simulink model "Sim_normboundsystem_simtest"  (Simulink 7.3)
settings: Solver=ode45  StartTime=0.0  StopTime=10  RelTol=1e-3
settings Model: Creator=MD710  LastModifiedBy=MD710
settings DebuggingCC: SaveWithParameterizedLinksMsg=none  MultiTaskDSMMsg=warning  MultiTaskCondExecSysMsg=none  FcnCallInpInsideContextMsg=Enable All  StrictBusMsg=None
settings HardwareCC: TargetHWDeviceType=32-bit Generic
settings RTWCC: IncludeERTFirstTime=on
settings GRTTargetCC: TargetFcnLib=ansi_tfl_tmw.mat

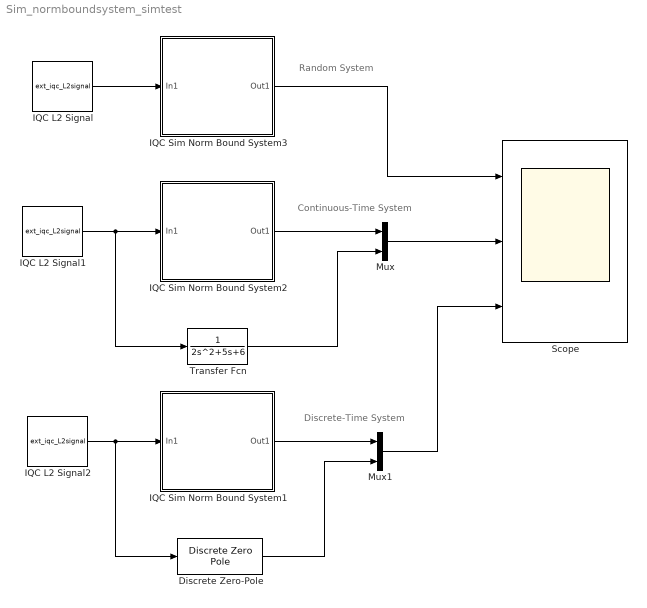
== system Sim_normboundsystem_simtest ==
  note: Random System
  note: Continuous-Time System
  note: Discrete-Time System
  Discrete Zero-Pole : DiscreteZeroPole  Zeros=[]  Poles=[0.3 -0.5]  Gain=1
  IQC L2 Signal : M-S-Function  FunctionName=ext_iqc_L2signal  Parameters=sig_size,sam_time,sig_type,tru_time,sig_amp,sig_fre,user_cus  mask(IQC L2 signal(ver:0.1)){sig_size=1, sam_time=0, sig_type=Sine wave, tru_time=10, sig_amp=1, sig_fre=1, user_cus='2*exp(3*t)'}
      mask prompts: sig_size "Signal Dimension:(Default: 1)"; sam_time "Sample Time:(Default: 0)"; sig_type "Signal Type:"; tru_time "Truncation Time:"; sig_amp "Maximum Amplitude:"; sig_fre "Frequency:"; user_cus "Custom:"
      mask help:
      | Important:
      | In IQC procedure step (as commond iqc_gain_tbx, the task is get
      | L2 gain value), regardless of the user to choose which option (ex sine...),
      | here regarded as generalized L2 signal.
      mask StyleString: edit,edit,popup(Step|Square wave|Sine wave|Custom|Random|External),edit,edit,edit,edit
      mask CallbackString: ||iqc_block_cho(gcb,'L2signal_type')||||
      mask TabNameString: Main,Main,Simulation,Simulation,Simulation,Simulation,Simulation
      mask Display: plot(0:0.1:10,[sin(0:0.1:6.2) zeros(1,38)])
  IQC L2 Signal1 : M-S-Function  FunctionName=ext_iqc_L2signal  Parameters=sig_size,sam_time,sig_type,tru_time,sig_amp,sig_fre,user_cus  mask(IQC L2 signal(ver:0.1)){sig_size=1, sam_time=0, sig_type=Sine wave, tru_time=10, sig_amp=1, sig_fre=1, user_cus='2*exp(3*t)'}
      mask prompts: sig_size "Signal Dimension:(Default: 1)"; sam_time "Sample Time:(Default: 0)"; sig_type "Signal Type:"; tru_time "Truncation Time:"; sig_amp "Maximum Amplitude:"; sig_fre "Frequency:"; user_cus "Custom:"
      mask help:
      | Important:
      | In IQC procedure step (as commond iqc_gain_tbx, the task is get
      | L2 gain value), regardless of the user to choose which option (ex sine...),
      | here regarded as generalized L2 signal.
      mask StyleString: edit,edit,popup(Step|Square wave|Sine wave|Custom|Random|External),edit,edit,edit,edit
      mask CallbackString: ||iqc_block_cho(gcb,'L2signal_type')||||
      mask TabNameString: Main,Main,Simulation,Simulation,Simulation,Simulation,Simulation
      mask Display: plot(0:0.1:10,[sin(0:0.1:6.2) zeros(1,38)])
  IQC L2 Signal2 : M-S-Function  FunctionName=ext_iqc_L2signal  Parameters=sig_size,sam_time,sig_type,tru_time,sig_amp,sig_fre,user_cus  mask(IQC L2 signal(ver:0.1)){sig_size=1, sam_time=1, sig_type=Sine wave, tru_time=10, sig_amp=1, sig_fre=1, user_cus='2*exp(3*t)'}
      mask prompts: sig_size "Signal Dimension:(Default: 1)"; sam_time "Sample Time:(Default: 0)"; sig_type "Signal Type:"; tru_time "Truncation Time:"; sig_amp "Maximum Amplitude:"; sig_fre "Frequency:"; user_cus "Custom:"
      mask help:
      | Important:
      | In IQC procedure step (as commond iqc_gain_tbx, the task is get
      | L2 gain value), regardless of the user to choose which option (ex sine...),
      | here regarded as generalized L2 signal.
      mask StyleString: edit,edit,popup(Step|Square wave|Sine wave|Custom|Random|External),edit,edit,edit,edit
      mask CallbackString: ||iqc_block_cho(gcb,'L2signal_type')||||
      mask TabNameString: Main,Main,Simulation,Simulation,Simulation,Simulation,Simulation
      mask Display: plot(0:0.1:10,[sin(0:0.1:6.2) zeros(1,38)])
  IQC Sim Norm Bound System1 : Subsystem  mask(IQC Sim Norm Bound System(ver:0.1)){sou_sys=Custom, num_inp=1, num_out=1, num_sta=3, upp_bou=1, sam_tim=1, cus='1/((z-0.3)*(z+0.5))', var_nam='', iqc1=on, iqc1_pole=[4], iqc1_out='', iqc2=on, lis_rel='out==iqc_ltigain(in)', swsystemtype=0, A=0, B=0, C=0, D=0, newsam_tim=0}
      mask prompts: sou_sys "Source of the system:(Default: Random)"; num_inp "The Number of Input:(Default: 1)"; num_out "The Number of Output:(Default: 1)"; num_sta "The Number of States:(Default: 1)"; upp_bou "Upper Bound of the Hinf-Norm:(default: 1)"; sam_tim "Sample Time:(Default: 0)"; cus "Custom: (Default: '1/(s+1)' or '1/(z+0.5)')"; var_nam "Variable Name:(Default: empty)"; iqc1 "iqc_ltiunmod(Input,Pole,Number Output,Upper Bound)"; iqc1_pole "Pole:(Default: [1])"; iqc1_out "Output Variable:(Default: empty)"; iqc2 "Custom IQC"; lis_rel "List of IQC Relationships:"; newsam_tim "Mask Parameter 19:"
      mask init:
      | swsystemtype=1;
      | A=randn(num_sta);
      | B=randn(num_sta,num_inp);
      | C=randn(num_out,num_sta);
      | D=randn(num_out,num_inp);
      | switch sou_sys
      |     case 1
      |         if sam_tim==0
      |             newsam_tim=1;
      |             A=A-(1+max(real(eig(A))))*eye(num_sta);
      |             G=ss(A,B,C,D);
      |             normG=norm(G,inf);
      |             G=G*upp_bou*rand/normG;
      |         elseif sam_tim>0
      |             newsam_tim=sam_tim;
      |             swsystemtype=2;
      |             A=A-(1+max(real(eig(A))))*eye(num_sta);
      |             G=ss(A,B,C,D);
      |             normG=norm(G,inf);
      |             G=G*upp_bou*rand/normG;
      |             G=c2d(G,sam_tim);
      |         else
      |             error(['sampletime set error'])
      |         end
      |     case 2
      |         s=tf('s');
      |         newsam_tim=1;
      |         if sam_tim>0
      |             newsam_tim=sam_tim;
      |             swsystemtype=2;
      |             z=tf('z',sam_tim);
      |         end
      |         if ischar(cus)
      |             eval(['G=ss(',cus,');']);
      |         else
      |             G=ss(cus);
      |         end
      | end
      | A=G.a;
      | B=G.b;
      | C=G.c;
      | D=G.d;
      mask Help: <a href="matlab:doc iqc_ltiunmod;">iqc_ltiunmod</a>
      mask StyleString: popup(Random|Custom),edit,edit,edit,edit,edit,edit,edit,checkbox,edit,edit,checkbox,edit,edit,edit,edit,edit,edit,edit
      mask CallbackString: iqc_block_cho(gcb,'sim_normboundsys_sou')||||||||iqc_block_cho(gcb,'sim_normboundsys_iqc1')|||iqc_block_cho(gcb,'sim_normboundsys_iqc2')|||||||
      mask TabNameString: Simulink Parameters,Simulink Parameters,Simulink Parameters,Simulink Parameters,Simulink Parameters,Simulink Parameters,Simulink Parameters,Simulink Parameters,Procedure Parameters,Procedure Parameters,Procedure Parameters,Procedure Parameters,Procedure Parameters,Simulink Parameters,Simulink Parameters,Simulink Parameters,Simulink Parameters,Simulink Parameters,Simulink Parameters
      mask Display: disp('\fontsize{14}||\Delta|| < k', 'texmode','on');
  IQC Sim Norm Bound System2 : Subsystem  mask(IQC Sim Norm Bound System(ver:0.1)){sou_sys=Custom, num_inp=1, num_out=1, num_sta=3, upp_bou=1, sam_tim=0, cus='1/(2*s*s+5*s+6)', var_nam='', iqc1=on, iqc1_pole=[4], iqc1_out='', iqc2=on, lis_rel='out==iqc_ltigain(in)', swsystemtype=0, A=0, B=0, C=0, D=0, newsam_tim=0}
      mask prompts: sou_sys "Source of the system:(Default: Random)"; num_inp "The Number of Input:(Default: 1)"; num_out "The Number of Output:(Default: 1)"; num_sta "The Number of States:(Default: 1)"; upp_bou "Upper Bound of the Hinf-Norm:(default: 1)"; sam_tim "Sample Time:(Default: 0)"; cus "Custom: (Default: '1/(s+1)' or '1/(z+0.5)')"; var_nam "Variable Name:(Default: empty)"; iqc1 "iqc_ltiunmod(Input,Pole,Number Output,Upper Bound)"; iqc1_pole "Pole:(Default: [1])"; iqc1_out "Output Variable:(Default: empty)"; iqc2 "Custom IQC"; lis_rel "List of IQC Relationships:"; newsam_tim "Mask Parameter 19:"
      mask init: same as Sim_normboundsystem_simtest/IQC Sim Norm Bound System1
      mask Help: <a href="matlab:doc iqc_ltiunmod;">iqc_ltiunmod</a>
      mask StyleString: popup(Random|Custom),edit,edit,edit,edit,edit,edit,edit,checkbox,edit,edit,checkbox,edit,edit,edit,edit,edit,edit,edit
      mask CallbackString: iqc_block_cho(gcb,'sim_normboundsys_sou')||||||||iqc_block_cho(gcb,'sim_normboundsys_iqc1')|||iqc_block_cho(gcb,'sim_normboundsys_iqc2')|||||||
      mask TabNameString: Simulink Parameters,Simulink Parameters,Simulink Parameters,Simulink Parameters,Simulink Parameters,Simulink Parameters,Simulink Parameters,Simulink Parameters,Procedure Parameters,Procedure Parameters,Procedure Parameters,Procedure Parameters,Procedure Parameters,Simulink Parameters,Simulink Parameters,Simulink Parameters,Simulink Parameters,Simulink Parameters,Simulink Parameters
      mask Display: disp('\fontsize{14}||\Delta|| < k', 'texmode','on');
  IQC Sim Norm Bound System3 : Subsystem  mask(IQC Sim Norm Bound System(ver:0.1)){sou_sys=Random, num_inp=1, num_out=1, num_sta=1, upp_bou=1, sam_tim=0, cus='1/(2*s*s+5*s+6)', var_nam='', iqc1=on, iqc1_pole=[4], iqc1_out='', iqc2=off, lis_rel='out==iqc_ltigain(in)', swsystemtype=0, A=0, B=0, C=0, D=0, newsam_tim=0}
      mask prompts: sou_sys "Source of the system:(Default: Random)"; num_inp "The Number of Input:(Default: 1)"; num_out "The Number of Output:(Default: 1)"; num_sta "The Number of States:(Default: 1)"; upp_bou "Upper Bound of the Hinf-Norm:(default: 1)"; sam_tim "Sample Time:(Default: 0)"; cus "Custom: (Default: '1/(s+1)' or '1/(z+0.5)')"; var_nam "Variable Name:(Default: empty)"; iqc1 "iqc_ltiunmod(Input,Pole,Number Output,Upper Bound)"; iqc1_pole "Pole:(Default: [1])"; iqc1_out "Output Variable:(Default: empty)"; iqc2 "Custom IQC"; lis_rel "List of IQC Relationships:"; newsam_tim "Mask Parameter 19:"
      mask init: same as Sim_normboundsystem_simtest/IQC Sim Norm Bound System1
      mask Help: <a href="matlab:doc iqc_ltiunmod;">iqc_ltiunmod</a>
      mask StyleString: popup(Random|Custom),edit,edit,edit,edit,edit,edit,edit,checkbox,edit,edit,checkbox,edit,edit,edit,edit,edit,edit,edit
      mask CallbackString: iqc_block_cho(gcb,'sim_normboundsys_sou')||||||||iqc_block_cho(gcb,'sim_normboundsys_iqc1')|||iqc_block_cho(gcb,'sim_normboundsys_iqc2')|||||||
      mask TabNameString: Simulink Parameters,Simulink Parameters,Simulink Parameters,Simulink Parameters,Simulink Parameters,Simulink Parameters,Simulink Parameters,Simulink Parameters,Procedure Parameters,Procedure Parameters,Procedure Parameters,Procedure Parameters,Procedure Parameters,Simulink Parameters,Simulink Parameters,Simulink Parameters,Simulink Parameters,Simulink Parameters,Simulink Parameters
      mask Display: disp('\fontsize{14}||\Delta|| < k', 'texmode','on');
  Mux : Mux  Inputs=2
  Mux1 : Mux  Inputs=2
  Scope : Scope  NumInputPorts=3
      settings: YMin=-0.175~-0.175~-1  YMax=0.175~0.175~1
  Transfer Fcn : TransferFcn  Denominator=[2 5 6]
  wires:
  IQC L2 Signal1/1 -> IQC Sim Norm Bound System2/1(In1), Transfer Fcn/1
  IQC L2 Signal/1 -> IQC Sim Norm Bound System3/1(In1)
  IQC Sim Norm Bound System2/1(Out1) -> Mux/1
  Transfer Fcn/1 -> Mux/2
  Mux/1 -> Scope/2
  IQC Sim Norm Bound System3/1(Out1) -> Scope/1
  IQC L2 Signal2/1 -> IQC Sim Norm Bound System1/1(In1), Discrete Zero-Pole/1
  IQC Sim Norm Bound System1/1(Out1) -> Mux1/1
  Discrete Zero-Pole/1 -> Mux1/2
  Mux1/1 -> Scope/3

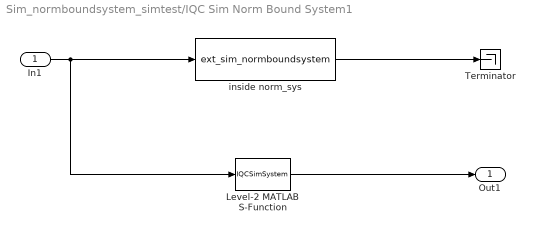
== system Sim_normboundsystem_simtest/IQC Sim Norm Bound System1 ==
  In1 : Inport
  Level-2 MATLAB S-Function : M-S-Function  FunctionName=IQCSimSystem  Parameters=A,B,C,D,sam_tim
  Terminator : Terminator
  inside norm_sys : M-S-Function  FunctionName=ext_sim_normboundsystem  Parameters=sou_sys,num_inp,num_out,num_sta,upp_bou,sam_tim,cus,var_nam,iqc1,iqc1_pole,iqc1_out,iqc2,lis_rel,swsystemtype,A,B,C,D,
  Out1 : Outport
  wires:
  inside norm_sys/1 -> Terminator/1
  In1/1 -> Level-2 MATLAB S-Function/1, inside norm_sys/1
  Level-2 MATLAB S-Function/1 -> Out1/1

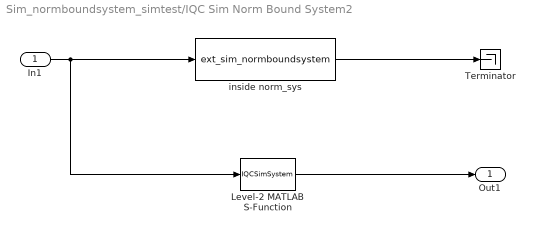
== system Sim_normboundsystem_simtest/IQC Sim Norm Bound System2 ==
  In1 : Inport
  Level-2 MATLAB S-Function : M-S-Function  FunctionName=IQCSimSystem  Parameters=A,B,C,D,sam_tim
  Terminator : Terminator
  inside norm_sys : M-S-Function  FunctionName=ext_sim_normboundsystem  Parameters=sou_sys,num_inp,num_out,num_sta,upp_bou,sam_tim,cus,var_nam,iqc1,iqc1_pole,iqc1_out,iqc2,lis_rel,swsystemtype,A,B,C,D,
  Out1 : Outport
  wires:
  Level-2 MATLAB S-Function/1 -> Out1/1
  In1/1 -> inside norm_sys/1, Level-2 MATLAB S-Function/1
  inside norm_sys/1 -> Terminator/1

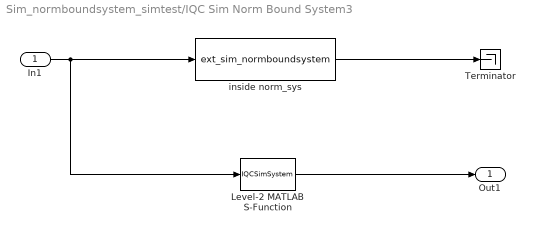
== system Sim_normboundsystem_simtest/IQC Sim Norm Bound System3 ==
  In1 : Inport
  Level-2 MATLAB S-Function : M-S-Function  FunctionName=IQCSimSystem  Parameters=A,B,C,D,sam_tim
  Terminator : Terminator
  inside norm_sys : M-S-Function  FunctionName=ext_sim_normboundsystem  Parameters=sou_sys,num_inp,num_out,num_sta,upp_bou,sam_tim,cus,var_nam,iqc1,iqc1_pole,iqc1_out,iqc2,lis_rel,swsystemtype,A,B,C,D,
  Out1 : Outport
  wires:
  inside norm_sys/1 -> Terminator/1
  In1/1 -> Level-2 MATLAB S-Function/1, inside norm_sys/1
  Level-2 MATLAB S-Function/1 -> Out1/1
